simulink model "TCDT"  (R2019b)
settings: Solver=ode4  StartTime=0.0  StopTime=tstop  FixedStep=tstep  RelTol=1e-3
settings Model: Creator=Ram Padmanabhan  LastModifiedBy=Ram Padmanabhan
settings DataIOCC: SaveOutput=off  SignalLogging=off  DSMLogging=off  SaveTime=off  ReturnWorkspaceOutputs=off

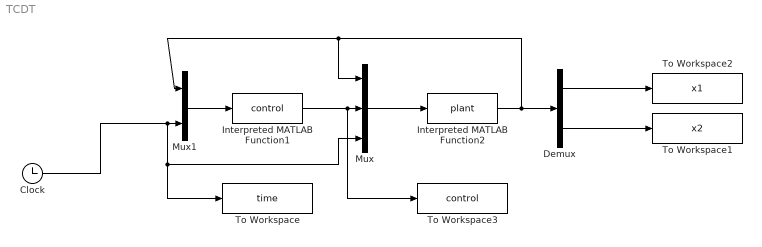
== system TCDT ==
  Clock : Clock
  Demux : Demux  Outputs=2
  Interpreted MATLAB Function1 : MATLABFcn  MATLABFcn=control  OutputDimensions=1
  Interpreted MATLAB Function2 : MATLABFcn  MATLABFcn=plant  OutputDimensions=2
  Mux : Mux  Inputs=3
  Mux1 : Mux  Inputs=2
  To Workspace : ToWorkspace  VariableName=time  SampleTime=-1
  To Workspace1 : ToWorkspace  VariableName=x2  SampleTime=-1
  To Workspace2 : ToWorkspace  VariableName=x1  SampleTime=-1
  To Workspace3 : ToWorkspace  VariableName=control  SampleTime=-1
  wires:
  Mux/1 -> Interpreted MATLAB Function2/1
  Interpreted MATLAB Function1/1 -> To Workspace3/1, Mux/2
  Mux1/1 -> Interpreted MATLAB Function1/1
  Clock/1 -> Mux/3, To Workspace/1, Mux1/2
  Demux/1 -> To Workspace2/1
  Demux/2 -> To Workspace1/1
  Interpreted MATLAB Function2/1 -> Mux1/1, Mux/1, Demux/1
